simulink model "drivetrainModel"  (R2023b)
settings: Solver=VariableStepAuto  StartTime=0.0  StopTime=ModelStopTime  RelTol=1e-3
undefined symbols (not defined in the file): K_us, steeringAngle_deg, wheelBase_m
libraries: sdl_lib x11, fl_lib x10, nesl_utility x4
settings Model: Creator=zuhai  LastModifiedBy=zuhai
settings SolverCC: MinimalZcImpactIntegration=on

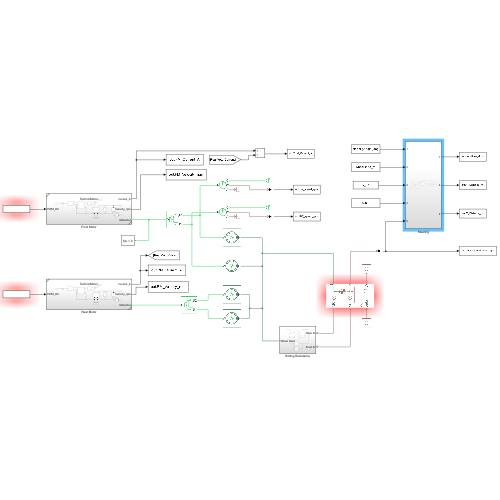
[thumbnail: Simulink's stored preview of the top-level diagram]
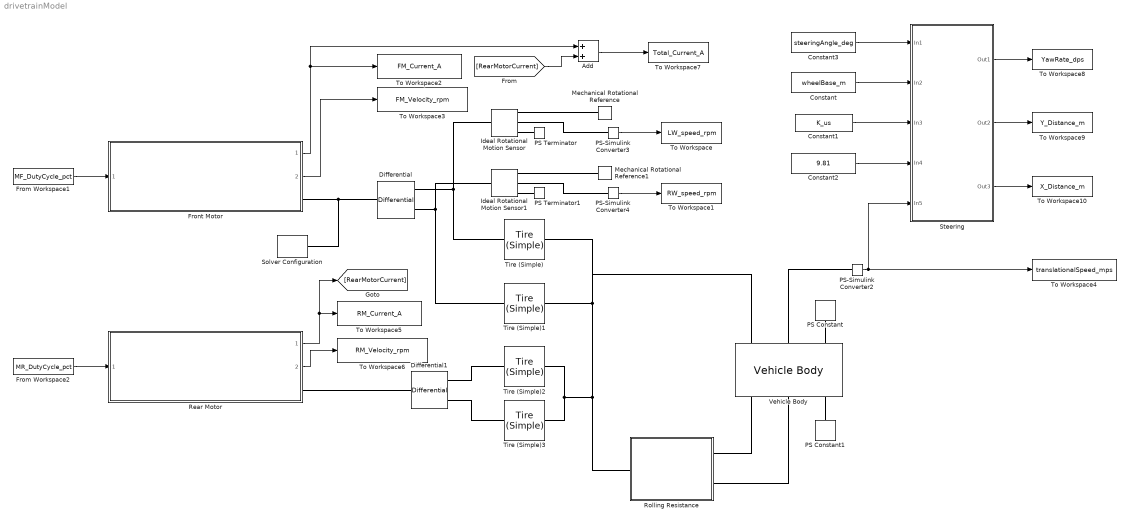
== system drivetrainModel ==
  Add : Sum
  Constant : Constant  Value=wheelBase_m
  Constant1 : Constant  Value=K_us
  Constant2 : Constant  Value=9.81
  Constant3 : Constant  Value=steeringAngle_deg
  Differential : sdl_lib/Gears/Differential  driveshaft_location=sdl.enum.differential_orientation.right  cd_ratio=n_diff  friction_model=sdl.enum.gear_friction.none  efficiency=[.85, .92]  temperature_TLU=[280, 300, 320] K  efficiency_ss_TLU=[.95, .9, .85]  efficiency_cd_TLU=[.95, .9, .85]  pwr_thr=[.001, .001] W  mu_visc=[0, 0] N*m*s/rad  model_inertia=simscape.enum.onoff.off  carrier_inertia=0.001 kg*m^2  planet_inertia=0.001 kg*m^2  thermal_mass=50 J/K  T_init=300 K
  Differential1 : sdl_lib/Gears/Differential  driveshaft_location=sdl.enum.differential_orientation.right  cd_ratio=n_diff  friction_model=sdl.enum.gear_friction.none  efficiency=[.85, .92]  temperature_TLU=[280, 300, 320] K  efficiency_ss_TLU=[.95, .9, .85]  efficiency_cd_TLU=[.95, .9, .85]  pwr_thr=[.001, .001] W  mu_visc=[0, 0] N*m*s/rad  model_inertia=simscape.enum.onoff.off  carrier_inertia=0.001 kg*m^2  planet_inertia=0.001 kg*m^2  thermal_mass=50 J/K  T_init=300 K
  From Workspace1 : FromWorkspace  VariableName=MF_DutyCycle_pct  SampleTime=0.1
  From Workspace2 : FromWorkspace  VariableName=MR_DutyCycle_pct  SampleTime=0.1
  Front Motor : Subsystem  ReferencedSubsystem=TechnicMotor
      settings: PortSchema="{\"entries\":[{\"content\":{\"sides\":[{\"content\":{\"connectorIds\":[\"In1\"]},\"type\":\"ConnectorPlacement.EquallySpacedRectSide\",\"uuid\":\"dbf9cfa3-e0fc-4ab8-aa03-97f57ea234b1\"},{\"content\":{\"connectorIds\":[\"Out1\",\"Out2\",\"LConn1\"],\"side\":\"RIGHT\"},\"type\":\"ConnectorPlacement.EquallySpacedRectSide\",\"uuid\":\"517209ad-f45f-45f4-8069-78c8dc36fc52\"},{\"content\":{\"side\":\"TOP\"},\"type\":\"ConnectorPlacement.EquallySpacedRectSide\",\"uuid\":\"9c5ebf90-c365-4f33-8958-3c576b7a8516\"}]},\"type\":\"ConnectorPlacement.EquallySpacedConnector\",\"uuid\":\"eb6a6e68-ae59-448c-beae-05913f52cb38\"}],\"packageUris\":[\"http://schema.mathworks.com/mf0/Connector/R2020b\"],\"version\":\"1.0\"}"
  Ideal Rotational Motion Sensor : fl_lib/Mechanical/Mechanical Sensors/Ideal Rotational Motion Sensor  reference=foundation.enum.MeasurementReference.difference  acceleration_port=false  velocity_port=true  position_port=true  wrap_angle=false  offset=0 rad
  Ideal Rotational Motion Sensor1 : fl_lib/Mechanical/Mechanical Sensors/Ideal Rotational Motion Sensor  reference=foundation.enum.MeasurementReference.difference  acceleration_port=false  velocity_port=true  position_port=true  wrap_angle=false  offset=0 rad
  Mechanical Rotational Reference : fl_lib/Mechanical/Rotational Elements/Mechanical Rotational Reference
  Mechanical Rotational Reference1 : fl_lib/Mechanical/Rotational Elements/Mechanical Rotational Reference
  PS Constant : fl_lib/Physical Signals/Sources/PS Constant  constant=0
  PS Constant1 : fl_lib/Physical Signals/Sources/PS Constant  constant=0
  PS Terminator : fl_lib/Physical Signals/Sinks/PS Terminator
  PS Terminator1 : fl_lib/Physical Signals/Sinks/PS Terminator
  PS-Simulink Converter2 : nesl_utility/PS-Simulink Converter  PhysicalDomain=network_engine_domain  SubClassName=ps_output  LeftPortType=input  RightPortType=output  PseudoPeriodic=off  Frequencies=[]  VectorFormat=inherit  Unit=m/s  AffineConversion=off
  PS-Simulink Converter3 : nesl_utility/PS-Simulink Converter  PhysicalDomain=network_engine_domain  SubClassName=ps_output  LeftPortType=input  RightPortType=output  PseudoPeriodic=off  Frequencies=[]  VectorFormat=inherit  Unit=rpm  AffineConversion=off
  PS-Simulink Converter4 : nesl_utility/PS-Simulink Converter  PhysicalDomain=network_engine_domain  SubClassName=ps_output  LeftPortType=input  RightPortType=output  PseudoPeriodic=off  Frequencies=[]  VectorFormat=inherit  Unit=rpm  AffineConversion=off
  Rear Motor : Subsystem  ReferencedSubsystem=TechnicMotor
      settings: PortSchema="{\"entries\":[{\"content\":{\"sides\":[{\"content\":{\"connectorIds\":[\"In1\"]},\"type\":\"ConnectorPlacement.EquallySpacedRectSide\",\"uuid\":\"dbf9cfa3-e0fc-4ab8-aa03-97f57ea234b1\"},{\"content\":{\"connectorIds\":[\"Out1\",\"Out2\",\"LConn1\"],\"side\":\"RIGHT\"},\"type\":\"ConnectorPlacement.EquallySpacedRectSide\",\"uuid\":\"517209ad-f45f-45f4-8069-78c8dc36fc52\"},{\"content\":{\"side\":\"TOP\"},\"type\":\"ConnectorPlacement.EquallySpacedRectSide\",\"uuid\":\"9c5ebf90-c365-4f33-8958-3c576b7a8516\"}]},\"type\":\"ConnectorPlacement.EquallySpacedConnector\",\"uuid\":\"eb6a6e68-ae59-448c-beae-05913f52cb38\"}],\"packageUris\":[\"http://schema.mathworks.com/mf0/Connector/R2020b\"],\"version\":\"1.0\"}"
  Rolling Resistance : Subsystem
  Solver Configuration : nesl_utility/Solver Configuration  PhysicalDomain=network_engine_domain  SubClassName=solver  LeftPortType=input  RightPortType=generic  Tones=[]  Harmonics=[]  SimulateNoise=off  Profile=off  UseLocalSampling=off  EnableSwitchedLinearOptims=on  FrequencyDomain=off  UseCCode=off  RelTol=0.001  AbsTol=0.001  MinStep=1e-09  ToWorkspace=off  RevertToSquareIcSolve=off  NumHomotopyIterations=100  PhasorMode=off  PhasorModeNumHarmonics=1  ConsistencySolver=NEWTON_XTOL_AFTER_FTOL  IndexReductionMethod=DerivativeReplacement  DoDC=off  ResidualTolerance=1e-09  ConsistencyTolSource=GLOBAL  ConsistencyAbsTol=0.001  ConsistencyRelTol=0.001  ConsistencyTolFactor=0.001  UseLocalSolver=off  LocalSolverChoice=NE_BACKWARD_EULER_ADVANCER  ResolveIndetEquations=on  FunctionEvalNumThread=1  LocalSolverSampleTime=0.001  DoFixedCost=off  MaxNonlinIter=3  MaxModeIter=2  ComputeImpulses=off  ImpulseIterations=2  LinearAlgebra=auto  LinearAlgebraNumThread=0  EquationFormulation=NE_TIME_EF  DelaysMemoryBudget=1024  AutomaticFiltering=on  FilteringTimeConstant=0.001  PartitionStorageMethod=AS_NEEDED  PartitionMemoryBudget=1024  PartitionMethod=ROBUST  MultibodyUseLocalSolver=off  MultibodyLocalSolverChoice=ODE1  MultibodyLocalSolverSampleTime=0.001
  Steering : Subsystem
  Tire (Simple){,1..3} (4 alike) : sdl_lib/Tires & Vehicles/Tire (Simple)  r_tire=TireRadius_m m  model_compliance=sdl.enum.compliance.on  stiffness=1e6 N/m  damping=1000 N*s/m  model_inertia=sdl.enum.model_inertia.off  tire_inertia=1 kg*m^2  initial_velocity=0 rad/s
      settings: InternalSimscapePortConfiguration="{\"Bottom\":[],\"Left\":[{\"id\":\"A\",\"label\":\"A\",\"type\":\"foundation.mechanical.rotational.rotational\"}],\"Right\":[{\"id\":\"H\",\"label\":\"H\",\"type\":\"foundation.mechanical.translational.translational\"}],\"Top\":[]}"
  To Workspace : ToWorkspace  VariableName=LW_speed_rpm  SaveFormat=Timeseries  SampleTime=-1
  To Workspace1 : ToWorkspace  VariableName=RW_speed_rpm  SaveFormat=Timeseries  SampleTime=-1
  To Workspace10 : ToWorkspace  VariableName=X_Distance_m  SaveFormat=Timeseries  SampleTime=-1
  To Workspace2 : ToWorkspace  VariableName=FM_Current_A  SaveFormat=Timeseries  SampleTime=-1
  To Workspace3 : ToWorkspace  VariableName=FM_Velocity_rpm  SaveFormat=Timeseries  SampleTime=-1
  To Workspace4 : ToWorkspace  VariableName=translationalSpeed_mps  SaveFormat=Timeseries  SampleTime=-1
  To Workspace5 : ToWorkspace  VariableName=RM_Current_A  SaveFormat=Timeseries  SampleTime=-1
  To Workspace6 : ToWorkspace  VariableName=RM_Velocity_rpm  SaveFormat=Timeseries  SampleTime=-1
  To Workspace7 : ToWorkspace  VariableName=Total_Current_A  SaveFormat=Timeseries  SampleTime=-1
  To Workspace8 : ToWorkspace  VariableName=YawRate_dps  SaveFormat=Timeseries  SampleTime=-1
  To Workspace9 : ToWorkspace  VariableName=Y_Distance_m  SaveFormat=Timeseries  SampleTime=-1
  Vehicle Body : sdl_lib/Tires & Vehicles/Vehicle Body  mass=vehicleMass_kg kg  n_w=2  x_f=0.132 m  x_r=0.105 m  y_c=0.075 m  mass_var=simscape.enum.onoff.off  g=9.81 m/s^2  liftoff_warning=simscape.enum.onoff.off  area=0.055^2 m^2  Cd=0.4  rho=1.18 kg/m^3  model_pitch=simscape.enum.onoff.off  inertia=4000 kg*m^2  suspension_model=sdl.enum.linearTLU.linear  k_f=1e4 N/m  b_f=1e4 N*s/m  k_r=1e4 N/m  b_r=1e4 N*s/m  k_f_TLU=[-2000, -1000, 0, 1000, 2000] N  x_f_TLU=[-.4, -.2, 0, .2, .4] m  b_f_TLU=[-200, -100, 0, 100, 200] N  v_f_TLU=[-4, -2, 0, 2, 4] m/s  k_r_TLU=[-2000, -1000, 0, 1000, 2000] N  x_r_TLU=[-.4, -.2, 0, .2, .4] m  b_r_TLU=[-200, -100, 0, 100, 200] N  v_r_TLU=[-4, -2, 0, 2, 4] m/s  interp_method=simscape.enum.interpolation.linear  extrap_method=simscape.enum.extrapolation.linear  model_hardstop=simscape.enum.onoff.off  upper_bound_f=.25 m  lower_bound_f=-.25 m  stop_k_f=1e6 N/m  stop_b_f=150 N*s/m  upper_bound_r=.25 m  lower_bound_r=-.25 m  stop_k_r=1e6 N/m  stop_b_r=150 N*s/m  initial_pitch=0 rad  initial_pitch_rate=0 rad/s  v_specify=off  v_priority=High  v=0 m/s  v_nominal_specify=off  v_nominal_unit=m/s  v_nominal_value=1
  wires:
  From Workspace1/1 -> Front Motor/1
  From Workspace2/1 -> Rear Motor/1
  PS-Simulink Converter3/1 -> To Workspace/1
  PS-Simulink Converter4/1 -> To Workspace1/1
  Front Motor/1 -> Add/1, To Workspace2/1
  Front Motor/2 -> To Workspace3/1
  PS-Simulink Converter2/1 -> Steering/5(In5), To Workspace4/1
  Rear Motor/1 -> [RearMotorCurrent], To Workspace5/1
  Rear Motor/2 -> To Workspace6/1
  [RearMotorCurrent] -> Add/2
  Add/1 -> To Workspace7/1
  Constant3/1 -> Steering/1(In1)
  Constant/1 -> Steering/2(In2)
  Constant1/1 -> Steering/3(In3)
  Constant2/1 -> Steering/4(In4)
  Steering/1(Out1) -> To Workspace8/1
  Steering/2(Out2) -> To Workspace9/1
  Steering/3(Out3) -> To Workspace10/1
  connections:
  Tire (Simple)2/RConn1 -- Tire (Simple)3/RConn1 -- Rolling Resistance/LConn1 -- Vehicle Body/LConn1 -- Tire (Simple)/RConn1 -- Tire (Simple)1/RConn1
  Differential1/RConn2 -- Tire (Simple)2/LConn1
  Differential1/RConn1 -- Tire (Simple)3/LConn1
  Vehicle Body/LConn2 -- PS-Simulink Converter2/LConn1
  Rear Motor/LConn1 -- Differential1/LConn1
  Mechanical Rotational Reference/LConn1 -- Ideal Rotational Motion Sensor/RConn1
  Ideal Rotational Motion Sensor/RConn2 -- PS-Simulink Converter3/LConn1
  Ideal Rotational Motion Sensor1/RConn2 -- PS-Simulink Converter4/LConn1
  Mechanical Rotational Reference1/LConn1 -- Ideal Rotational Motion Sensor1/RConn1
  PS Terminator/LConn1 -- Ideal Rotational Motion Sensor/RConn3
  PS Terminator1/LConn1 -- Ideal Rotational Motion Sensor1/RConn3
  Front Motor/LConn1 -- Solver Configuration/RConn1 -- Differential/LConn1
  Differential/RConn2 -- Ideal Rotational Motion Sensor/LConn1 -- Tire (Simple)/LConn1
  Differential/RConn1 -- Tire (Simple)1/LConn1 -- Ideal Rotational Motion Sensor1/LConn1
  PS Constant/RConn1 -- Vehicle Body/LConn3
  PS Constant1/RConn1 -- Vehicle Body/RConn3
  Vehicle Body/RConn1 -- Rolling Resistance/RConn1
  Vehicle Body/RConn2 -- Rolling Resistance/RConn2

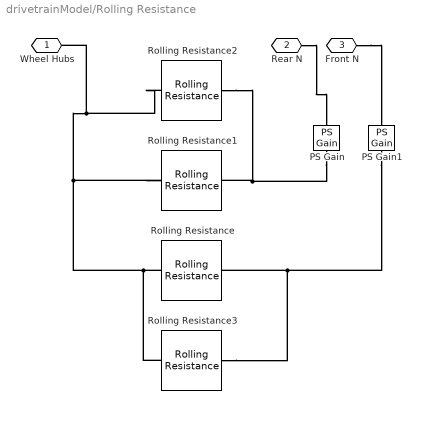
== system drivetrainModel/Rolling Resistance ==
  PS Gain : fl_lib/Physical Signals/Functions/PS Gain  gain=0.5
  PS Gain1 : fl_lib/Physical Signals/Functions/PS Gain  gain=0.5
  Rolling Resistance{,1..3} (4 alike) : sdl_lib/Tires & Vehicles/Tire Subcomponents/Rolling Resistance  model=sdl.enum.rollingResistanceParameterization.constant  coeff=f_r  p_tire=250e3 Pa  alpha=-0.003  beta=0.97  coeff_a=84e-4  coeff_b=6.2e-4 s/m  coeff_c=1.6e-4 s^2/m^2  p_tire0=240e3 Pa  fz0=4000 N  vH0=16 m/s  q_Sy=[.0082, 0, .0014, .001, 0, 0, 1.08, -.5]  lmy=1  v_thr=0.001 m/s
      settings: InternalSimscapePortConfiguration="{\"Bottom\":[],\"Left\":[{\"id\":\"N\",\"label\":\"N\",\"type\":\"input\"}],\"Right\":[{\"id\":\"H\",\"label\":\"H\",\"type\":\"foundation.mechanical.translational.translational\"}],\"Top\":[]}"
  Wheel Hubs : PMIOPort  Side=Left
  Rear N : PMIOPort  Port=2  Side=Right
  Front N : PMIOPort  Port=3  Side=Right
  connections:
  Rolling Resistance2/RConn1 -- Wheel Hubs/RConn1 -- Rolling Resistance3/RConn1 -- Rolling Resistance/RConn1 -- Rolling Resistance1/RConn1
  PS Gain1/RConn1 -- Rolling Resistance3/LConn1 -- Rolling Resistance/LConn1
  PS Gain/RConn1 -- Rolling Resistance2/LConn1 -- Rolling Resistance1/LConn1
  Front N/RConn1 -- PS Gain1/LConn1
  Rear N/RConn1 -- PS Gain/LConn1

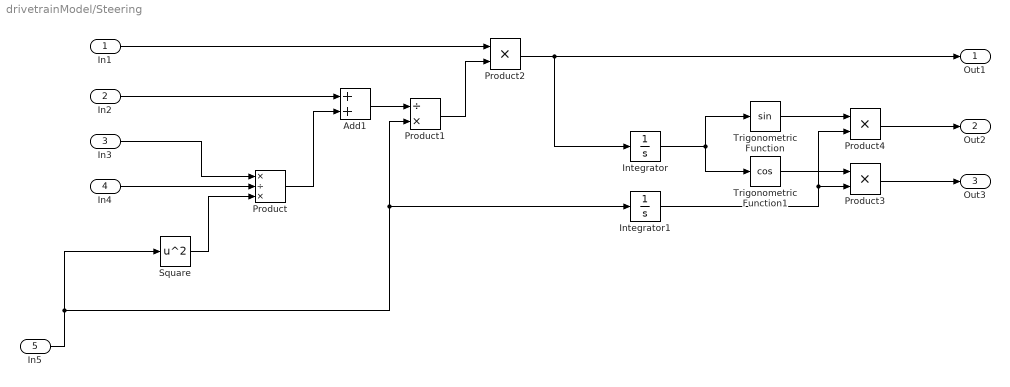
== system drivetrainModel/Steering ==
  In1 : Inport
  In2 : Inport  Port=2
  In3 : Inport  Port=3
  In4 : Inport  Port=4
  In5 : Inport  Port=5
  Add1 : Sum
  Integrator : Integrator
  Integrator1 : Integrator
  Product : Product  Inputs=*/*
  Product1 : Product  Inputs=/*
  Product2 : Product
  Product3 : Product
  Product4 : Product
  Square : Math  Operator=square
  Trigonometric Function : Trigonometry
  Trigonometric Function1 : Trigonometry  Operator=cos
  Out1 : Outport
  Out2 : Outport  Port=2
  Out3 : Outport  Port=3
  wires:
  Integrator1/1 -> Product4/2, Product3/2
  Product4/1 -> Out2/1
  In3/1 -> Product/1
  Trigonometric Function/1 -> Product4/1
  Square/1 -> Product/3
  Product2/1 -> Out1/1, Integrator/1
  Integrator/1 -> Trigonometric Function1/1, Trigonometric Function/1
  Product/1 -> Add1/2
  Add1/1 -> Product1/1
  Trigonometric Function1/1 -> Product3/1
  In4/1 -> Product/2
  Product3/1 -> Out3/1
  Product1/1 -> Product2/2
  In5/1 -> Integrator1/1, Product1/2, Square/1
  In2/1 -> Add1/1
  In1/1 -> Product2/1
